simulink model "pole_regulator_simulink_model"  (R2020b)
settings: Solver=VariableStepAuto  StartTime=0.0  StopTime=100  RelTol=1e-3
values from neighbouring files (symbols this model uses):
  C = [1 c_1 c_2 c_3 ]    [pole_regulator.m]
  D = [d_0  d_1 ]    [pole_regulator.m]
  Kr = polyval(P,1) / polyval(B,1)    [pole_regulator.m]
undefined symbols (not defined in the file or in its folder): GpDen, GpNum
settings Model: Creator=BadAzz Dan  LastModifiedBy=BadAzz Dan

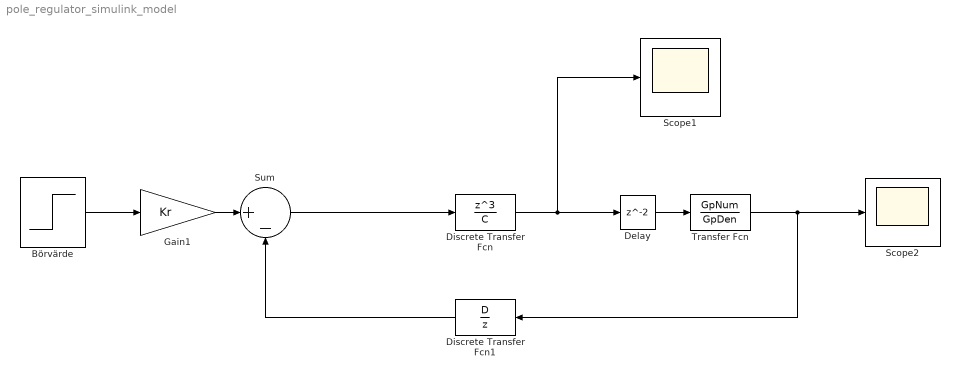
== system pole_regulator_simulink_model ==
  Börvärde : Step  Time=0  SampleTime=1
  Delay : Delay  SampleTime=1
  Discrete Transfer Fcn : DiscreteTransferFcn  Numerator=[1 0 0 0]  Denominator=C  SampleTime=1
  Discrete Transfer Fcn1 : DiscreteTransferFcn  Numerator=D  Denominator=[1 0]  SampleTime=1
  Gain1 : Gain  Gain=Kr
  Scope1 : Scope
  Scope2 : Scope
  Sum : Sum  Inputs=|+-
  Transfer Fcn : TransferFcn  Numerator=GpNum  Denominator=GpDen
  wires:
  Börvärde/1 -> Gain1/1
  Sum/1 -> Discrete Transfer Fcn/1
  Discrete Transfer Fcn1/1 -> Sum/2
  Gain1/1 -> Sum/1
  Discrete Transfer Fcn/1 -> Scope1/1, Delay/1
  Delay/1 -> Transfer Fcn/1
  Transfer Fcn/1 -> Discrete Transfer Fcn1/1, Scope2/1
